simulink model "check_RLS_estimated_model"  (R2023a)
settings: Solver=FixedStepDiscrete  StartTime=0.0  StopTime=0  FixedStep=TimeStep_MPC  RelTol=1e-3
undefined symbols (not defined in the file): EKF_u_num, EKF_y_num
settings Model: DataDictionary=BallAndPlate_system_data.sldd  Creator=tshintai  LastModifiedBy=tshintai
settings OptimizationCC: ReuseModelBlockBuffer=off
settings DebuggingCC: ParameterPrecisionLossMsg=none
settings ModelReferenceCC: EnableRefExpFcnMdlSchedulingChecks=on

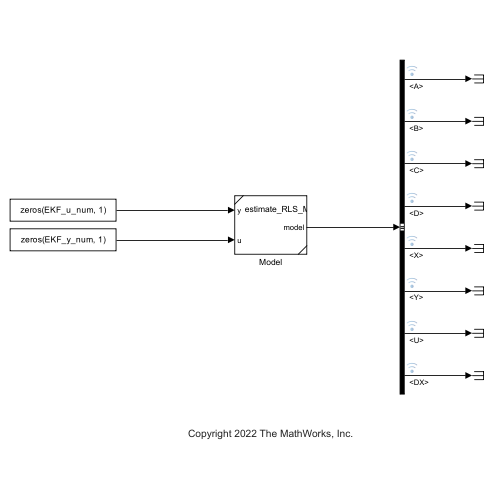
[thumbnail: Simulink's stored preview of the top-level diagram]
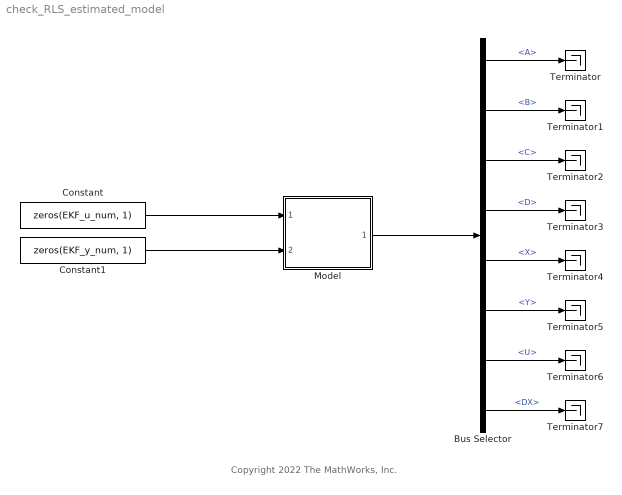
== system check_RLS_estimated_model ==
  note: Copyright 2022 The MathWorks, Inc.
  Bus Selector : BusSelector  OutputSignals=A,B,C,D,X,Y,U,DX
  Constant : Constant  Value=zeros(EKF_u_num, 1)  OutDataTypeStr=single
  Constant1 : Constant  Value=zeros(EKF_y_num, 1)  OutDataTypeStr=single
  Model : Subsystem  ReferencedSubsystem=estimate_RLS_MPC_Model
  Terminator{,1..7} (8 alike) : Terminator
  wires:
  Bus Selector/3 -> Terminator2/1  "<C>"
  Bus Selector/8 -> Terminator7/1  "<DX>"
  Bus Selector/2 -> Terminator1/1  "<B>"
  Bus Selector/4 -> Terminator3/1  "<D>"
  Bus Selector/6 -> Terminator5/1  "<Y>"
  Bus Selector/7 -> Terminator6/1  "<U>"
  Bus Selector/1 -> Terminator/1  "<A>"
  Model/1 -> Bus Selector/1
  Constant/1 -> Model/1
  Constant1/1 -> Model/2
  Bus Selector/5 -> Terminator4/1  "<X>"
